simulink model "Uloha11"  (R2017b)
settings: Solver=VariableStepAuto  StartTime=0.0  StopTime=10.0  RelTol=1e-3
values from neighbouring files (symbols this model uses):
  P1 = [1 0 -p2 -p3]    [Uloha7.m]    (also in ulo.m = [1 0 -p1 -p2]; uloha6.m)
  Q = [q0 q1 q2]    [Uloha7.m]    (also in ulo.m; uloha6.m)
settings Model: Creator=jan.sedivy  LastModifiedBy=jan.sedivy

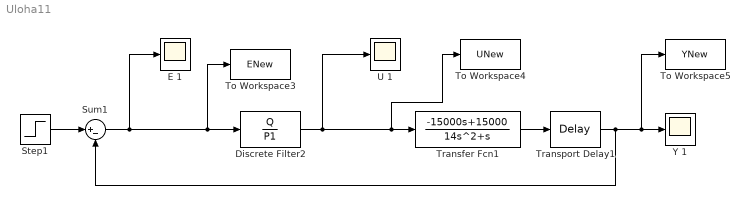
== system Uloha11 ==
  Discrete Filter2 : DiscreteFilter  Numerator=Q  Denominator=P1  SampleTime=1
  E 1 : Scope
  Step1 : Step  Time=0  SampleTime=0
  Sum1 : Sum  Inputs=|+-
  To Workspace3 : ToWorkspace  VariableName=ENew  SaveFormat=Timeseries  SampleTime=-1
  To Workspace4 : ToWorkspace  VariableName=UNew  SaveFormat=Timeseries  SampleTime=-1
  To Workspace5 : ToWorkspace  VariableName=YNew  SaveFormat=Timeseries  SampleTime=-1
  Transfer Fcn1 : TransferFcn  Numerator=[-15000 15000]  Denominator=[14 1 0]
  Transport Delay1 : TransportDelay
  U 1 : Scope
  Y 1 : Scope
  wires:
  Discrete Filter2/1 -> U 1/1, To Workspace4/1, Transfer Fcn1/1
  Transport Delay1/1 -> Sum1/2, To Workspace5/1, Y 1/1
  Step1/1 -> Sum1/1
  Transfer Fcn1/1 -> Transport Delay1/1
  Sum1/1 -> Discrete Filter2/1, To Workspace3/1, E 1/1
